simulink library "coordinate_transform_lib"  (R2017b)
settings: Solver=VariableStepAuto  StartTime=0.0  StopTime=10.0  RelTol=1e-3
settings Model: Creator=Máté  LastModifiedBy=Máté

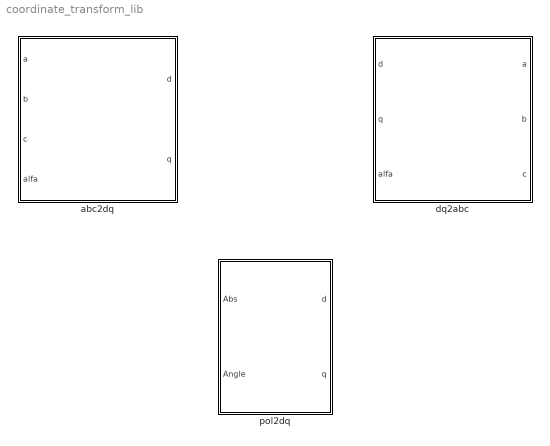
== system coordinate_transform_lib ==
  "abc2dq " : Subsystem
  dq2abc : Subsystem
  pol2dq : Subsystem

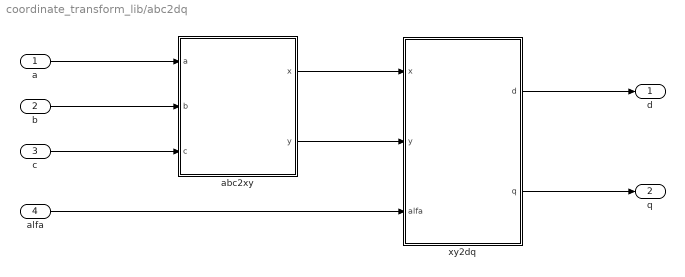
== system coordinate_transform_lib/abc2dq  ==
  a : Inport
  b : Inport  Port=2
  c : Inport  Port=3
  alfa : Inport  Port=4
  abc2xy : Subsystem
  xy2dq : Subsystem
  d : Outport
  q : Outport  Port=2
  wires:
  a/1 -> abc2xy/1(a)
  abc2xy/1(x) -> xy2dq/1(x)
  xy2dq/2(q) -> q/1
  xy2dq/1(d) -> d/1
  c/1 -> abc2xy/3(c)
  b/1 -> abc2xy/2(b)
  abc2xy/2(y) -> xy2dq/2(y)
  alfa/1 -> xy2dq/3("alfa ")

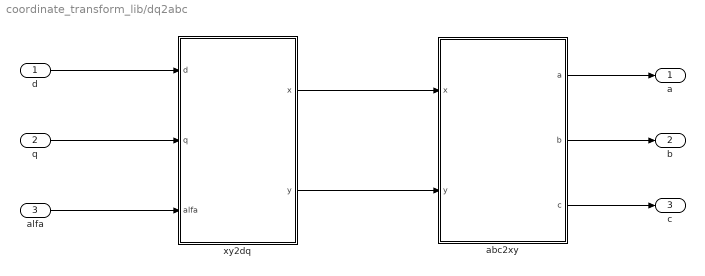
== system coordinate_transform_lib/dq2abc ==
  d : Inport
  q : Inport  Port=2
  alfa : Inport  Port=3
  abc2xy : Subsystem
  xy2dq : Subsystem
  a : Outport
  b : Outport  Port=2
  c : Outport  Port=3
  wires:
  xy2dq/2(y) -> abc2xy/2(y)
  xy2dq/1(x) -> abc2xy/1(x)
  alfa/1 -> xy2dq/3("alfa ")
  q/1 -> xy2dq/2(q)
  d/1 -> xy2dq/1(d)
  abc2xy/1(a) -> a/1
  abc2xy/2(b) -> b/1
  abc2xy/3(c) -> c/1

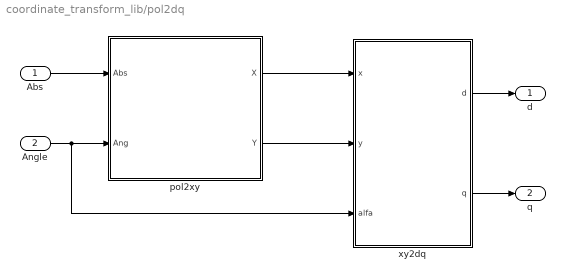
== system coordinate_transform_lib/pol2dq ==
  Abs : Inport
  Angle : Inport  Port=2
  pol2xy : Subsystem
  xy2dq : Subsystem
  d : Outport
  q : Outport  Port=2
  wires:
  pol2xy/1(X) -> xy2dq/1(x)
  xy2dq/1(d) -> d/1
  xy2dq/2(q) -> q/1
  Angle/1 -> xy2dq/3("alfa "), pol2xy/2(Ang)
  Abs/1 -> pol2xy/1(Abs)
  pol2xy/2(Y) -> xy2dq/2(y)

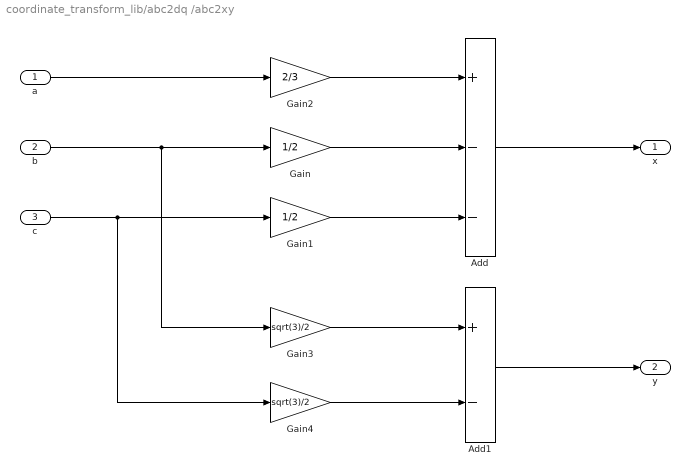
== system coordinate_transform_lib/abc2dq /abc2xy ==
  a : Inport
  b : Inport  Port=2
  c : Inport  Port=3
  Add : Sum  Inputs=+--
  Add1 : Sum  Inputs=+-
  Gain : Gain  Gain=1/2
  Gain1 : Gain  Gain=1/2
  Gain2 : Gain  Gain=2/3
  Gain3 : Gain  Gain=sqrt(3)/2
  Gain4 : Gain  Gain=sqrt(3)/2
  x : Outport
  y : Outport  Port=2
  wires:
  a/1 -> Gain2/1
  Gain2/1 -> Add/1
  b/1 -> Gain3/1, Gain/1
  c/1 -> Gain4/1, Gain1/1
  Gain/1 -> Add/2
  Gain1/1 -> Add/3
  Add/1 -> x/1
  Gain3/1 -> Add1/1
  Gain4/1 -> Add1/2
  Add1/1 -> y/1

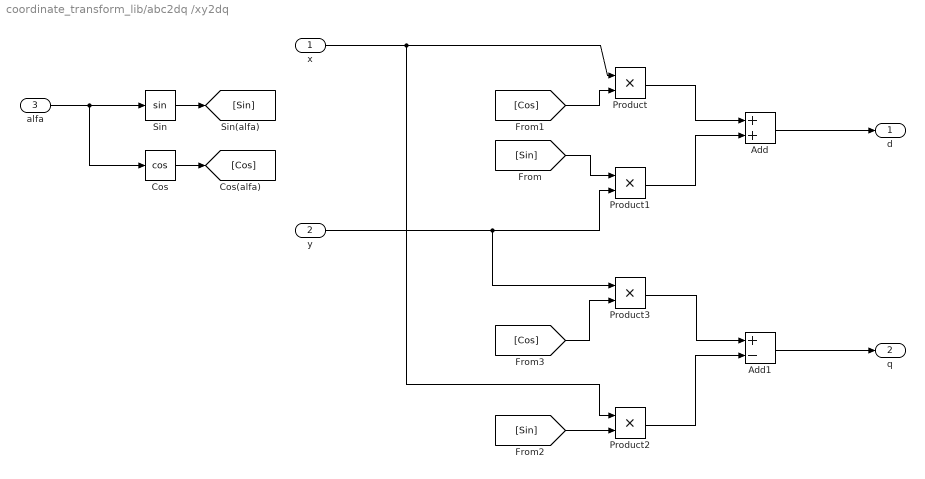
== system coordinate_transform_lib/abc2dq /xy2dq ==
  x : Inport
  y : Inport  Port=2
  "alfa " : Inport  Port=3
  Add : Sum
  Add1 : Sum  Inputs=+-
  Cos : Trigonometry  Operator=cos
  Product{,1..3} (4 alike) : Product
  Sin : Trigonometry
  d : Outport
  q : Outport  Port=2
  wires:
  "alfa "/1 -> Cos/1, Sin/1
  Sin/1 -> [Sin]
  Cos/1 -> [Cos]
  x/1 -> Product2/1, Product/1
  [Cos] -> Product/2
  Product/1 -> Add/1
  [Sin] -> Product1/1
  y/1 -> Product3/1, Product1/2
  Product1/1 -> Add/2
  Add/1 -> d/1
  Add1/1 -> q/1
  [Sin] -> Product2/2
  Product2/1 -> Add1/2
  [Cos] -> Product3/2
  Product3/1 -> Add1/1

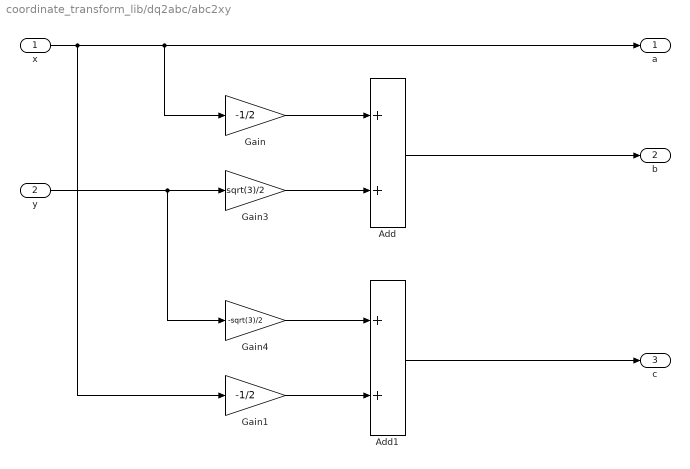
== system coordinate_transform_lib/dq2abc/abc2xy ==
  x : Inport
  y : Inport  Port=2
  Add : Sum
  Add1 : Sum
  Gain : Gain  Gain=-1/2
  Gain1 : Gain  Gain=-1/2
  Gain3 : Gain  Gain=sqrt(3)/2
  Gain4 : Gain  Gain=-sqrt(3)/2
  a : Outport
  b : Outport  Port=2
  c : Outport  Port=3
  wires:
  x/1 -> Gain1/1, Gain/1, a/1
  Add/1 -> b/1
  Gain/1 -> Add/1
  Gain3/1 -> Add/2
  y/1 -> Gain4/1, Gain3/1
  Gain4/1 -> Add1/1
  Gain1/1 -> Add1/2
  Add1/1 -> c/1

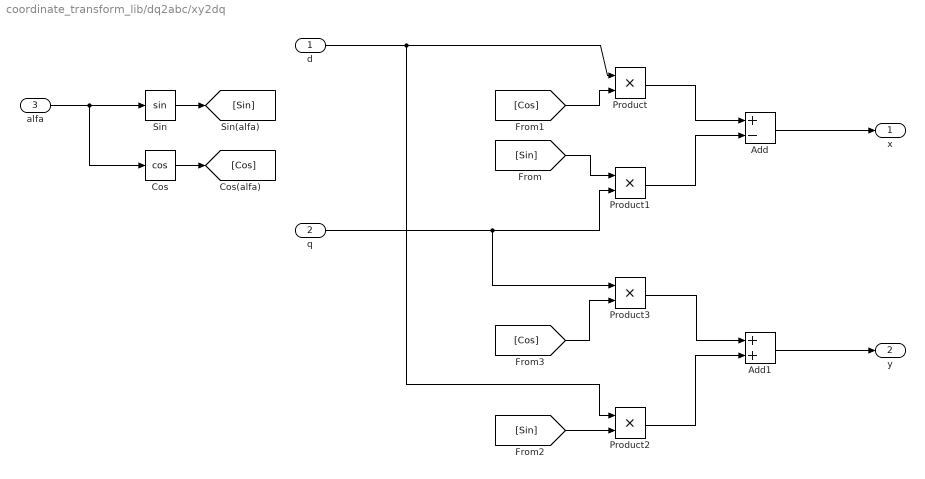
== system coordinate_transform_lib/dq2abc/xy2dq ==
  d : Inport
  q : Inport  Port=2
  "alfa " : Inport  Port=3
  Add : Sum  Inputs=+-
  Add1 : Sum
  Cos : Trigonometry  Operator=cos
  Product{,1..3} (4 alike) : Product
  Sin : Trigonometry
  x : Outport
  y : Outport  Port=2
  wires:
  Product3/1 -> Add1/1
  [Cos] -> Product3/2
  Product2/1 -> Add1/2
  [Sin] -> Product2/2
  Add1/1 -> y/1
  Add/1 -> x/1
  Product1/1 -> Add/2
  q/1 -> Product1/2, Product3/1
  [Sin] -> Product1/1
  Product/1 -> Add/1
  [Cos] -> Product/2
  d/1 -> Product/1, Product2/1
  Cos/1 -> [Cos]
  Sin/1 -> [Sin]
  "alfa "/1 -> Sin/1, Cos/1

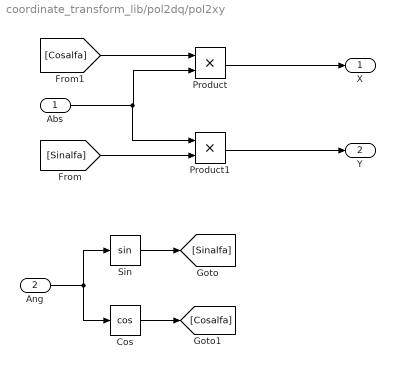
== system coordinate_transform_lib/pol2dq/pol2xy ==
  Abs : Inport
  Ang : Inport  Port=2
  Cos : Trigonometry  Operator=cos
  Product : Product
  Product1 : Product
  Sin : Trigonometry
  X : Outport
  Y : Outport  Port=2
  wires:
  Ang/1 -> Cos/1, Sin/1
  Sin/1 -> [Sinalfa]
  Cos/1 -> [Cosalfa]
  Abs/1 -> Product1/1, Product/2
  Product/1 -> X/1
  Product1/1 -> Y/1
  [Cosalfa] -> Product/1
  [Sinalfa] -> Product1/2

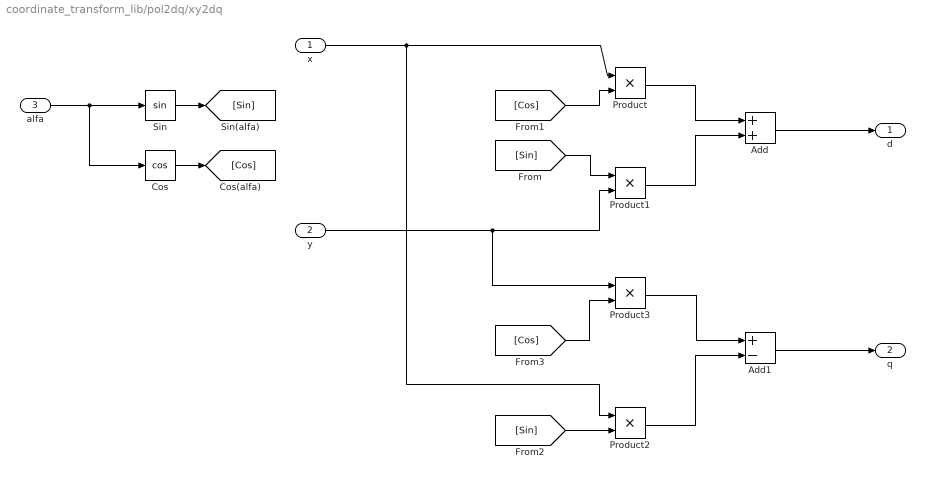
== system coordinate_transform_lib/pol2dq/xy2dq ==
  x : Inport
  y : Inport  Port=2
  "alfa " : Inport  Port=3
  Add : Sum
  Add1 : Sum  Inputs=+-
  Cos : Trigonometry  Operator=cos
  Product{,1..3} (4 alike) : Product
  Sin : Trigonometry
  d : Outport
  q : Outport  Port=2
  wires:
  Product3/1 -> Add1/1
  [Cos] -> Product3/2
  Product2/1 -> Add1/2
  [Sin] -> Product2/2
  Add1/1 -> q/1
  Add/1 -> d/1
  Product1/1 -> Add/2
  y/1 -> Product1/2, Product3/1
  [Sin] -> Product1/1
  Product/1 -> Add/1
  [Cos] -> Product/2
  x/1 -> Product/1, Product2/1
  Cos/1 -> [Cos]
  Sin/1 -> [Sin]
  "alfa "/1 -> Sin/1, Cos/1
